simulink model "figure_1_6"  (R2026a)
settings: Solver=ode5  FixedStep=1e-4
settings Model: Creator=yagmu  LastModifiedBy=yagmu

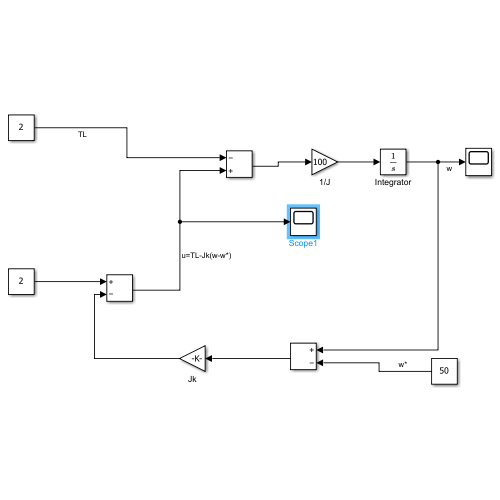
[thumbnail: Simulink's stored preview of the top-level diagram]
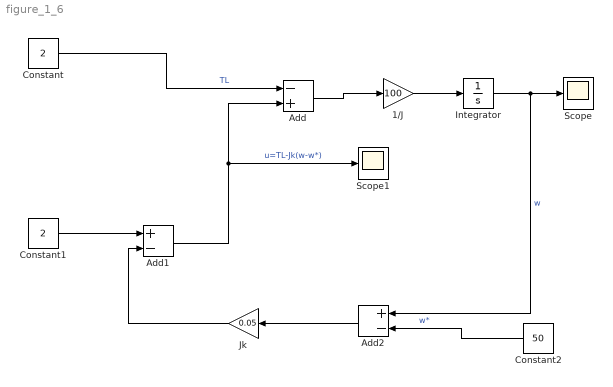
== system figure_1_6 ==
  1/J : Gain  Gain=100
  Add : Sum  Inputs=-+
  Add1 : Sum  Inputs=+-
  Add2 : Sum  Inputs=+-
  Constant : Constant  Value=2
  Constant1 : Constant  Value=2
  Constant2 : Constant  Value=50
  Integrator : Integrator
  Jk : Gain  Gain=0.05
  Scope : Scope
      settings: ActiveDisplayYMinimum=40  ActiveDisplayYMaximum=60
  Scope1 : Scope
      settings: ActiveDisplayYMinimum=1.6875000000003997  ActiveDisplayYMaximum=4.8124999999999556
  wires:
  Constant/1 -> Add/1  "TL"
  Add/1 -> 1/J/1
  1/J/1 -> Integrator/1
  Integrator/1 -> Scope/1, Add2/1  "w"
  Constant1/1 -> Add1/1
  Constant2/1 -> Add2/2  "w*"
  Add1/1 -> Scope1/1, Add/2  "u=TL-Jk(w-w*)"
  Jk/1 -> Add1/2
  Add2/1 -> Jk/1
